simulink model "observador"  (R2020b)
settings: Solver=VariableStepAuto  StartTime=0.0  StopTime=40  RelTol=1e-3
undefined symbols (not defined in the file): Agorro, Gss2, L
settings Model: Creator=andre  LastModifiedBy=andre

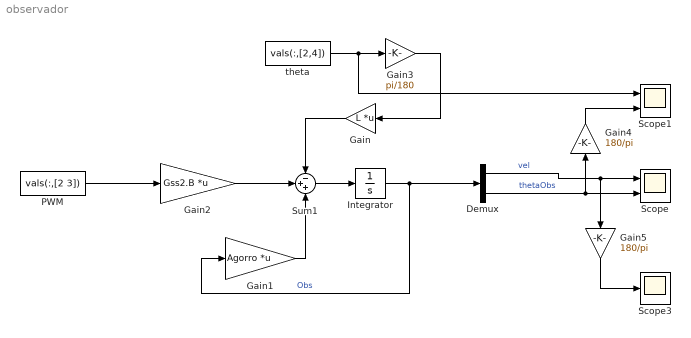
== system observador ==
  Demux : Demux  Outputs=2
  Gain : Gain  Gain=L  Multiplication=Matrix(K*u)
  Gain1 : Gain  Gain=Agorro  Multiplication=Matrix(K*u)
  Gain2 : Gain  Gain=Gss2.B  Multiplication=Matrix(K*u)
  Gain3 : Gain  Gain=pi/180
  Gain4 : Gain  Gain=180/pi
  Gain5 : Gain  Gain=180/pi
  Integrator : Integrator
  PWM : FromWorkspace  VariableName=vals(:,[2 3])  SampleTime=0.0025
  Scope : Scope  NumInputPorts=2
  Scope1 : Scope  NumInputPorts=2
  Scope3 : Scope
  Sum1 : Sum  Inputs=-++
  theta : FromWorkspace  VariableName=vals(:,[2,4])  SampleTime=0.0025
  wires:
  Gain/1 -> Sum1/1
  PWM/1 -> Gain2/1
  Gain1/1 -> Sum1/3
  Gain2/1 -> Sum1/2
  Sum1/1 -> Integrator/1
  Integrator/1 -> Demux/1, Gain1/1  "Obs"
  theta/1 -> Scope1/1, Gain3/1
  Demux/1 -> Gain5/1, Scope/1  "vel"
  Demux/2 -> Scope/2, Gain4/1  "thetaObs"
  Gain3/1 -> Gain/1
  Gain4/1 -> Scope1/2
  Gain5/1 -> Scope3/1
